simulink model "old_plant_2015B"  (R2015b)
settings: Solver=ode1  StartTime=0.0  StopTime=sim_run  FixedStep=0.001  RelTol=1e-3
InitFcn:
  | [g,m1,T1,f_1s,f_1k,m2,l,f_2k,M_sp,f_1k_lin,f_2k_lin,k1,k2] =...
  |     set_system_parameters();
undefined symbols (not defined in the file): DiscIntNeverNeededParam, f_1k, f_1k_lin, f_1s, f_2k, f_2k_lin, g, k1, k2, l, m1, m2, M_sp, sgn, Standard_Devices, UDP_Protocol, zh_step
libraries: sldrtlib x4, dspnetwork x2
settings Model: Creator=Anony  LastModifiedBy=Anony

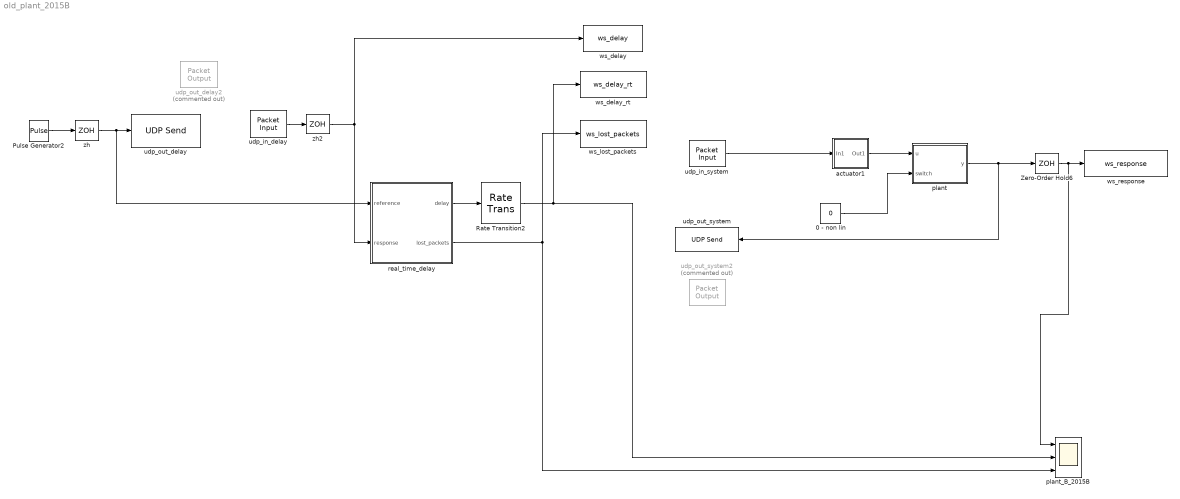
== system old_plant_2015B ==
  0 - non lin : Constant  Value=0
  Pulse Generator2 : DiscretePulseGenerator  PulseType=Time based  Period=0.1
  Rate Transition2 : RateTransition  OutPortSampleTimeOpt=Inherit
  Zero-Order Hold6 : ZeroOrderHold  SampleTime=zh_step
  actuator1 : Subsystem
  plant : Subsystem
  plant_B_2015B : Scope  NumInputPorts=3
  real_time_delay : Subsystem
  udp_in_delay : sldrtlib/Packet Input  SampleTime=0.001  MaxMissedTicks=inf  ShowMissedTicks=off  YieldWhenWaiting=off  DrvName=Standard_Devices/UDP_Protocol  DrvAddress=20000  DrvOptions=[2468394761 20000]  PacketSize=8  DataTypes='double'  ShowReady=off  ShowError=off  PacketID=1  ByteOrder=1  ShowTimestamp=off
      settings: AttributesFormatString=Standard Devices\nUDP Protocol [6982h]
  udp_in_system : sldrtlib/Packet Input  SampleTime=0.001  MaxMissedTicks=inf  ShowMissedTicks=off  YieldWhenWaiting=off  DrvName=Standard_Devices/UDP_Protocol  DrvAddress=20500  DrvOptions=[2468394761 20500]  PacketSize=8  DataTypes='double'  ShowReady=off  ShowError=off  PacketID=1  ByteOrder=1  ShowTimestamp=off
      settings: AttributesFormatString=Standard Devices\nUDP Protocol [6B76h]
  udp_out_delay : dspnetwork/UDP Send  remoteURL='147.32.183.9'  remotePort=21000  localURL='0.0.0.0'  localPortSource=Automatically determine  localPort=27000  sampletime=-1  separateLengthPort=0
  udp_out_delay2 : sldrtlib/Packet Output  Commented=on  SampleTime=0.01  MaxMissedTicks=inf  ShowMissedTicks=off  YieldWhenWaiting=off  DrvName=Standard_Devices/UDP_Protocol  DrvAddress=21000  DrvOptions=[2468394756 21000]  PacketSize=8  DataTypes='double'  ShowReady=off  ShowError=off  PacketID=1  ByteOrder=1  InitialValue=[]  FinalValue=[]
  udp_out_system : dspnetwork/UDP Send  remoteURL='147.32.183.9'  remotePort=21500  localURL='0.0.0.0'  localPortSource=Automatically determine  localPort=27000  sampletime=-1  separateLengthPort=0
  udp_out_system2 : sldrtlib/Packet Output  Commented=on  SampleTime=0.01  MaxMissedTicks=inf  ShowMissedTicks=off  YieldWhenWaiting=off  DrvName=Standard_Devices/UDP_Protocol  DrvAddress=21500  DrvOptions=[2468394761 21500]  PacketSize=8  DataTypes='double'  ShowReady=off  ShowError=off  PacketID=1  ByteOrder=1  InitialValue=[]  FinalValue=[]
  ws_delay : ToWorkspace  VariableName=ws_delay  SaveFormat=Timeseries  SampleTime=zh_step
  ws_delay_rt : ToWorkspace  VariableName=ws_delay_rt  SaveFormat=Timeseries  SampleTime=zh_step
  ws_lost_packets : ToWorkspace  VariableName=ws_lost_packets  SaveFormat=Timeseries  SampleTime=zh_step
  ws_response : ToWorkspace  VariableName=ws_response  SaveFormat=Timeseries  SampleTime=zh_step
  zh : ZeroOrderHold  SampleTime=zh_step
  zh2 : ZeroOrderHold  SampleTime=zh_step
  wires:
  plant/1(y) -> udp_out_system/1, Zero-Order Hold6/1
  0 - non lin/1 -> plant/2(switch)
  actuator1/1(Out1) -> plant/1(u)
  udp_in_system/1 -> actuator1/1(In1)
  udp_in_delay/1 -> zh2/1
  zh2/1 -> real_time_delay/2(response), ws_delay/1
  zh/1 -> udp_out_delay/1, real_time_delay/1(reference)
  real_time_delay/2(lost_packets) -> plant_B_2015B/3, ws_lost_packets/1
  real_time_delay/1(delay) -> Rate Transition2/1
  Pulse Generator2/1 -> zh/1
  Rate Transition2/1 -> ws_delay_rt/1, plant_B_2015B/2
  Zero-Order Hold6/1 -> plant_B_2015B/1, ws_response/1

== system old_plant_2015B/actuator1 ==
  In1 : Inport
  V > N1 : Gain  Gain=4
  mv > V1 : Gain  Gain=1000
  Out1 : Outport
  wires:
  In1/1 -> mv > V1/1
  mv > V1/1 -> V > N1/1
  V > N1/1 -> Out1/1

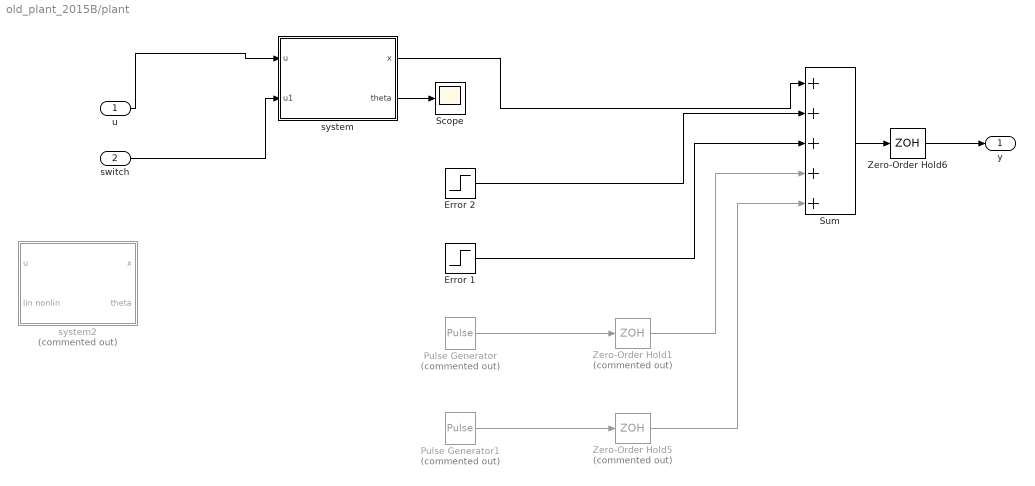
== system old_plant_2015B/plant ==
  u : Inport
  switch : Inport  Port=2
  Error 1 : Step  Time=15  After=0.02  SampleTime=0
  Error 2 : Step  Time=10  After=-0.02  SampleTime=0
  Pulse Generator : DiscretePulseGenerator  Commented=on  PulseType=Time based  Amplitude=0.3  Period=3  PulseWidth=5  PhaseDelay=15
  Pulse Generator1 : DiscretePulseGenerator  Commented=on  PulseType=Time based  Amplitude=-0.18  Period=3  PulseWidth=5  PhaseDelay=25
  Scope : Scope
  Sum : Sum  Inputs=|+++++
  Zero-Order Hold1 : ZeroOrderHold  Commented=on  SampleTime=zh_step
  Zero-Order Hold5 : ZeroOrderHold  Commented=on  SampleTime=zh_step
  Zero-Order Hold6 : ZeroOrderHold  SampleTime=zh_step
  system : Subsystem
  system2 : Subsystem  Commented=on
  y : Outport
  wires:
  system/2(theta) -> Scope/1
  switch/1 -> system/2(u1)
  u/1 -> system/1(u)
  Zero-Order Hold5/1 -> Sum/5
  Pulse Generator1/1 -> Zero-Order Hold5/1
  Zero-Order Hold1/1 -> Sum/4
  Pulse Generator/1 -> Zero-Order Hold1/1
  Error 1/1 -> Sum/3
  system/1(x) -> Sum/1
  Error 2/1 -> Sum/2
  Sum/1 -> Zero-Order Hold6/1
  Zero-Order Hold6/1 -> y/1

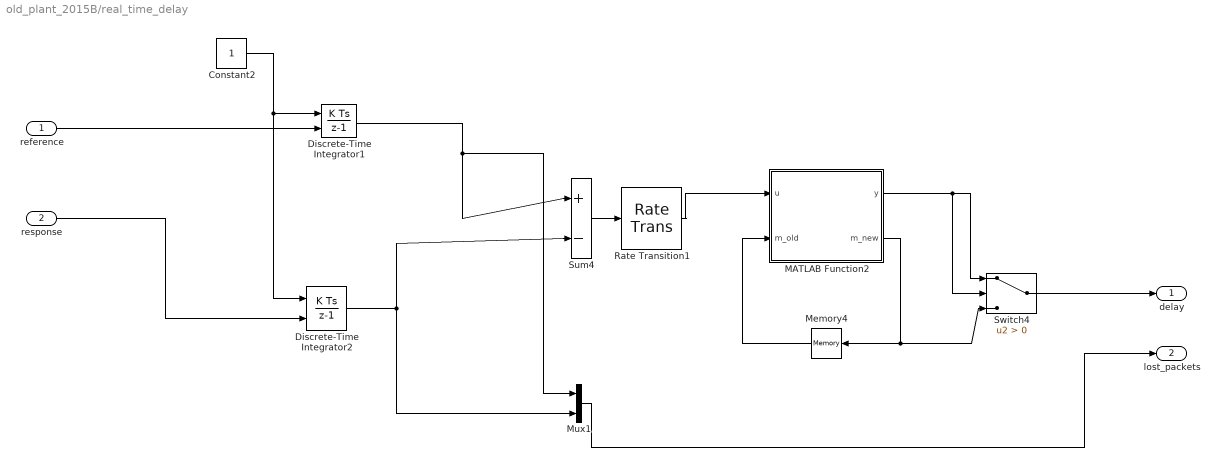
== system old_plant_2015B/real_time_delay ==
  reference : Inport
  response : Inport  Port=2
  Constant2 : Constant
  Discrete-Time Integrator1 : DiscreteIntegrator  ExternalReset=rising  InitialConditionSetting=State (most efficient)  SampleTime=zh_step  ICPrevOutput=DiscIntNeverNeededParam  ICPrevScaledInput=DiscIntNeverNeededParam
  Discrete-Time Integrator2 : DiscreteIntegrator  ExternalReset=rising  InitialConditionSetting=State (most efficient)  SampleTime=zh_step  ICPrevOutput=DiscIntNeverNeededParam  ICPrevScaledInput=DiscIntNeverNeededParam
  MATLAB Function2 : MATLAB Function  TreatAsAtomicUnit=on
  Memory4 : Memory
  Mux1 : Mux  Inputs=2
  Rate Transition1 : RateTransition  OutPortSampleTimeOpt=Inherit
  Sum4 : Sum  Inputs=|+-
  Switch4 : Switch  Criteria=u2 > Threshold
  delay : Outport
  lost_packets : Outport  Port=2
  wires:
  Discrete-Time Integrator1/1 -> Mux1/1, Sum4/1
  reference/1 -> Discrete-Time Integrator1/2
  Constant2/1 -> Discrete-Time Integrator2/1, Discrete-Time Integrator1/1
  response/1 -> Discrete-Time Integrator2/2
  Switch4/1 -> delay/1
  MATLAB Function2/2(m_new) -> Memory4/1, Switch4/3
  Memory4/1 -> MATLAB Function2/2(m_old)
  Discrete-Time Integrator2/1 -> Mux1/2, Sum4/2
  Mux1/1 -> lost_packets/1
  MATLAB Function2/1(y) -> Switch4/2, Switch4/1
  Sum4/1 -> Rate Transition1/1
  Rate Transition1/1 -> MATLAB Function2/1(u)

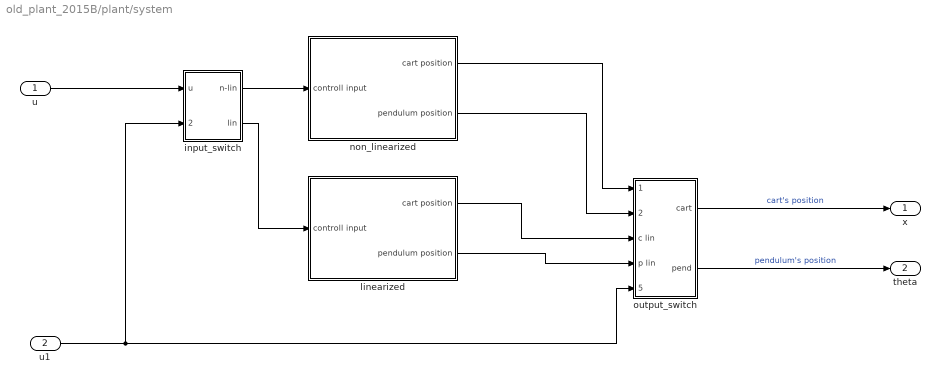
== system old_plant_2015B/plant/system ==
  u : Inport
  u1 : Inport  Port=2
  input_switch : Subsystem
  linearized : Subsystem
  non_linearized : Subsystem
  output_switch : Subsystem
  x : Outport
  theta : Outport  Port=2
  wires:
  u1/1 -> input_switch/2(switch), output_switch/5(switch)
  u/1 -> input_switch/1(u)
  output_switch/2(pend) -> theta/1  "pendulum's position"
  linearized/2("pendulum position ") -> output_switch/4(p lin)
  linearized/1(cart position) -> output_switch/3(c lin)
  non_linearized/2("pendulum position ") -> output_switch/2(p n-lin)
  non_linearized/1(cart position) -> output_switch/1(c n-lin)
  output_switch/1(cart) -> x/1  "cart's position"
  input_switch/2("lin ") -> linearized/1(controll input)
  input_switch/1(n-lin) -> non_linearized/1(controll input)

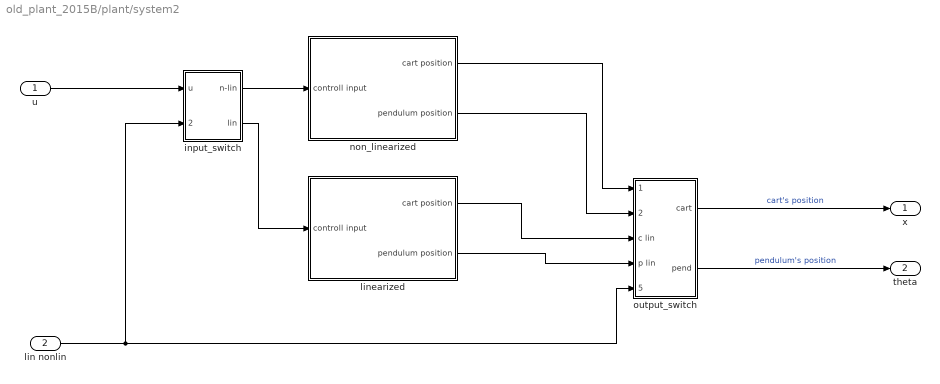
== system old_plant_2015B/plant/system2 ==
  u : Inport
  lin nonlin : Inport  Port=2
  input_switch : Subsystem
  linearized : Subsystem
  non_linearized : Subsystem
  output_switch : Subsystem
  x : Outport
  theta : Outport  Port=2
  wires:
  input_switch/1(n-lin) -> non_linearized/1(controll input)
  input_switch/2("lin ") -> linearized/1(controll input)
  output_switch/1(cart) -> x/1  "cart's position"
  non_linearized/1(cart position) -> output_switch/1(c n-lin)
  non_linearized/2("pendulum position ") -> output_switch/2(p n-lin)
  linearized/1(cart position) -> output_switch/3(c lin)
  linearized/2("pendulum position ") -> output_switch/4(p lin)
  output_switch/2(pend) -> theta/1  "pendulum's position"
  u/1 -> input_switch/1(u)
  lin nonlin/1 -> output_switch/5(switch), input_switch/2(switch)

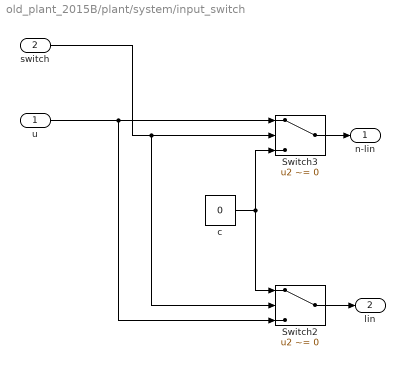
== system old_plant_2015B/plant/system/input_switch ==
  u : Inport
  switch : Inport  Port=2
  Switch2 : Switch  Criteria=u2 ~= 0  Threshold=1
  Switch3 : Switch  Criteria=u2 ~= 0  Threshold=1
  c : Constant  Value=0
  n-lin : Outport
  "lin " : Outport  Port=2
  wires:
  switch/1 -> Switch3/2, Switch2/2
  u/1 -> Switch3/1, Switch2/3
  Switch2/1 -> "lin "/1
  Switch3/1 -> n-lin/1
  c/1 -> Switch2/1, Switch3/3

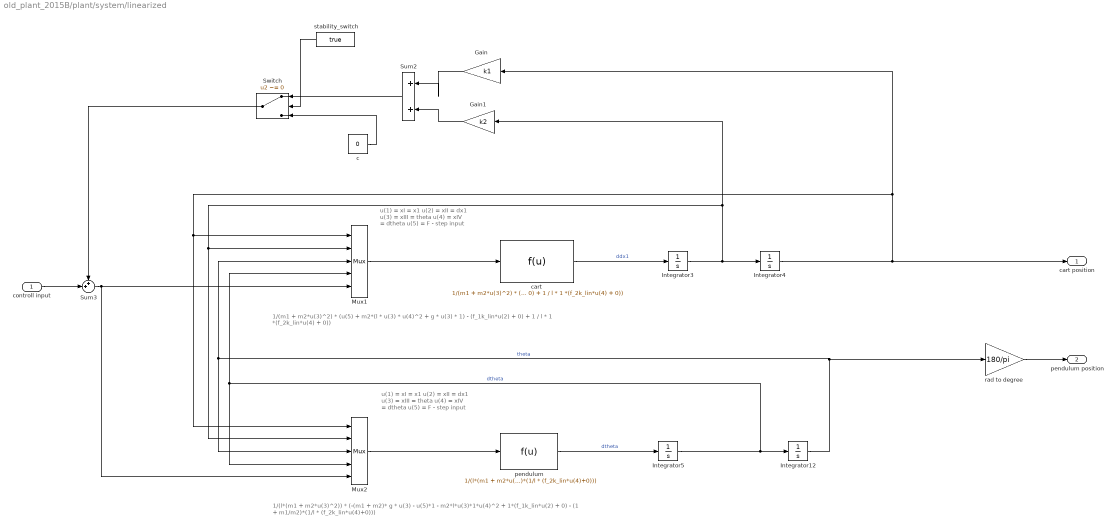
== system old_plant_2015B/plant/system/linearized ==
  note: 1/(l*(m1 + m2*u(3)^2)) * (-(m1 + m2)* g * u(3) - u(5)*1 - m2*l*u(3)*1*u(4)^2 + 1*(f_1k_lin*u(2) + 0) - (1 + m1/m2)*(1/l * (f_2k_lin*u(4)+0)))
  note: 1/(m1 + m2*u(3)^2) * (u(5) + m2*(l * u(3) * u(4)^2 + g * u(3) * 1) - (f_1k_lin*u(2) + 0) + 1 / l * 1 *(f_2k_lin*u(4) + 0))
  note: u(1) = xI = x1
      | u(2) = xII = dx1
      | u(3) = xIII = theta
      | u(4) = xIV = dtheta
      | u(5) = F - step input
  note: u(1) = xI = x1
      | u(2) = xII = dx1
      | u(3) = xIII = theta
      | u(4) = xIV = dtheta
      | u(5) = F - step input
  controll input : Inport
  Gain : Gain  Gain=k1
  Gain1 : Gain  Gain=k2
  Integrator{3..5,12} (4 alike) : Integrator
  Mux1 : Mux  Inputs=5
  Mux2 : Mux  Inputs=5
  Sum2 : Sum  Inputs=|++
  Sum3 : Sum  Inputs=++|
  Switch : Switch  Criteria=u2 ~= 0
  c : Constant  Value=0
  cart : Fcn  Expr=1/(m1 + m2*u(3)^2) * (u(5) + m2*(l * u(3) * u(4)^2 + g * u(3) * 1) - (f_1k_lin*u(2) + 0) + 1 / l * 1 *(f_2k_lin*u(4) + 0))
  "pendulum " : Fcn  Expr=1/(l*(m1 + m2*u(3)^2)) * (-(m1 + m2)* g * u(3) - u(5)*1 - m2*l*u(3)*1*u(4)^2 + 1*(f_1k_lin*u(2) + 0) - (1 + m1/m2)*(1/l * (f_2k_lin*u(4)+0)))
  rad to degree : Gain  Gain=180/pi
  stability_switch : Constant  Value=true
  cart position : Outport
  "pendulum position " : Outport  Port=2
  wires:
  stability_switch/1 -> Switch/2
  Switch/1 -> Sum3/1
  Sum2/1 -> Switch/1
  Sum3/1 -> Mux1/5, Mux2/5
  controll input/1 -> Sum3/2
  Gain1/1 -> Sum2/2
  Gain/1 -> Sum2/1
  Integrator4/1 -> cart position/1, Mux2/1, Mux1/1, Gain/1
  Integrator3/1 -> Integrator4/1, Mux2/2, Mux1/2, Gain1/1
  cart/1 -> Integrator3/1  "ddx1"
  Mux2/1 -> "pendulum "/1
  "pendulum "/1 -> Integrator5/1  "dtheta"
  Integrator5/1 -> Integrator12/1, Mux1/4, Mux2/4  "dtheta"
  Integrator12/1 -> rad to degree/1, Mux1/3, Mux2/3  "theta"
  Mux1/1 -> cart/1
  rad to degree/1 -> "pendulum position "/1
  c/1 -> Switch/3

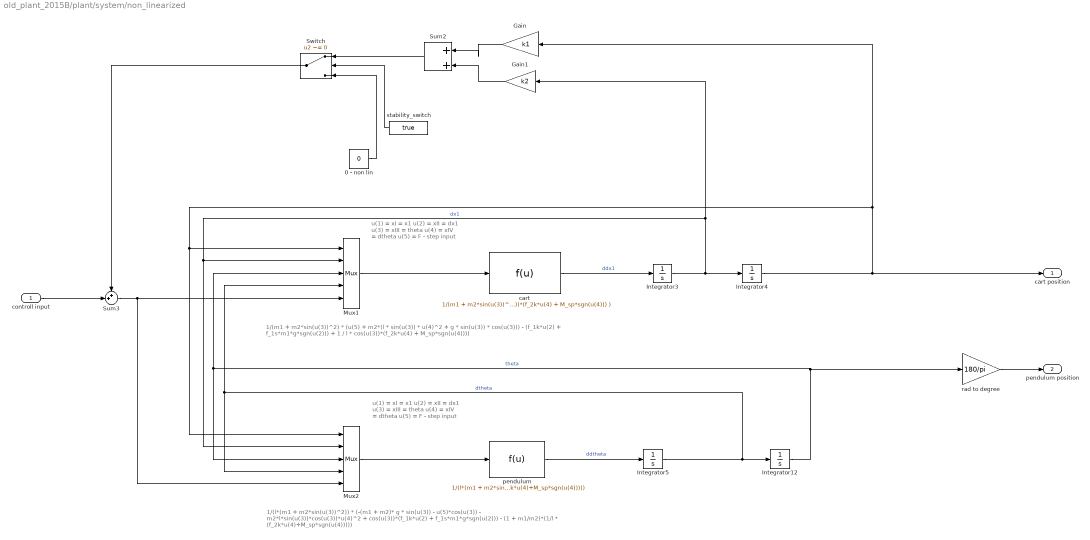
== system old_plant_2015B/plant/system/non_linearized ==
  note: u(1) = xI = x1
      | u(2) = xII = dx1
      | u(3) = xIII = theta
      | u(4) = xIV = dtheta
      | u(5) = F - step input
  note: u(1) = xI = x1
      | u(2) = xII = dx1
      | u(3) = xIII = theta
      | u(4) = xIV = dtheta
      | u(5) = F - step input
  note: 1/(m1 + m2*sin(u(3))^2) * (u(5) + m2*(l * sin(u(3)) * u(4)^2 + g * sin(u(3)) * cos(u(3))) - (f_1k*u(2) + f_1s*m1*g*sgn(u(2))) + 1 / l * cos(u(3))*(f_2k*u(4) + M_sp*sgn(u(4))))
  note: 1/(l*(m1 + m2*sin(u(3))^2)) * (-(m1 + m2)* g * sin(u(3)) - u(5)*cos(u(3)) - m2*l*sin(u(3))*cos(u(3))*u(4)^2 + cos(u(3))*(f_1k*u(2) + f_1s*m1*g*sgn(u(2))) - (1 + m1/m2)*(1/l * (f_2k*u(4)+M_sp*sgn(u(4)))))
  controll input : Inport
  0 - non lin : Constant  Value=0
  Gain : Gain  Gain=k1
  Gain1 : Gain  Gain=k2
  Integrator{3..5,12} (4 alike) : Integrator
  Mux1 : Mux  Inputs=5
  Mux2 : Mux  Inputs=5
  Sum2 : Sum  Inputs=|++
  Sum3 : Sum  Inputs=++|
  Switch : Switch  Criteria=u2 ~= 0
  cart : Fcn  Expr=1/(m1 + m2*sin(u(3))^2) * (u(5) + m2*(l * sin(u(3)) * u(4)^2 + g * sin(u(3)) * cos(u(3))) - (f_1k*u(2) + f_1s*m1*g*sgn(u(2))) + 1 / l * cos(u(3))*(f_2k*u(4) + M_sp*sgn(u(4))) )
  "pendulum " : Fcn  Expr=1/(l*(m1 + m2*sin(u(3))^2)) * (-(m1 + m2)* g * sin(u(3)) - u(5)*cos(u(3)) - m2*l*sin(u(3))*cos(u(3))*u(4)^2 + cos(u(3))*(f_1k*u(2) + f_1s*m1*g*sgn(u(2))) - (1 + m1/m2)*(1/l * (f_2k*u(4)+M_sp*sgn(u(4)))))
  rad to degree : Gain  Gain=180/pi
  stability_switch : Constant  Value=true
  cart position : Outport
  "pendulum position " : Outport  Port=2
  wires:
  Sum3/1 -> Mux1/5, Mux2/5
  controll input/1 -> Sum3/2
  stability_switch/1 -> Switch/2
  Switch/1 -> Sum3/1
  Sum2/1 -> Switch/1
  Gain1/1 -> Sum2/2
  Gain/1 -> Sum2/1
  Integrator4/1 -> Mux1/1, Mux2/1, Gain/1, cart position/1
  rad to degree/1 -> "pendulum position "/1
  Mux1/1 -> cart/1
  Integrator12/1 -> Mux2/3, Mux1/3, rad to degree/1  "theta"
  Integrator3/1 -> Mux1/2, Mux2/2, Gain1/1, Integrator4/1  "dx1"
  Integrator5/1 -> Mux2/4, Mux1/4, Integrator12/1  "dtheta"
  "pendulum "/1 -> Integrator5/1  "ddtheta"
  Mux2/1 -> "pendulum "/1
  cart/1 -> Integrator3/1  "ddx1"
  0 - non lin/1 -> Switch/3

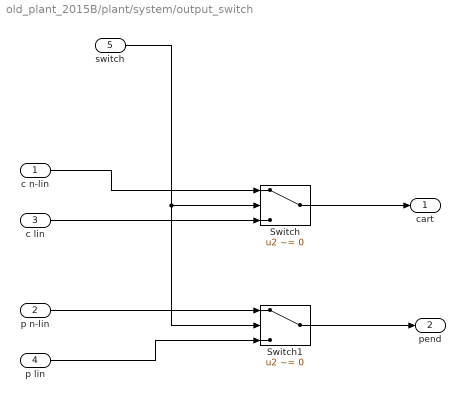
== system old_plant_2015B/plant/system/output_switch ==
  c n-lin : Inport
  p n-lin : Inport  Port=2
  c lin : Inport  Port=3
  p lin : Inport  Port=4
  switch : Inport  Port=5
  Switch : Switch  Criteria=u2 ~= 0  Threshold=1
  Switch1 : Switch  Criteria=u2 ~= 0  Threshold=1
  cart : Outport
  pend : Outport  Port=2
  wires:
  p n-lin/1 -> Switch1/1
  c n-lin/1 -> Switch/1
  Switch1/1 -> pend/1
  c lin/1 -> Switch/3
  Switch/1 -> cart/1
  p lin/1 -> Switch1/3
  switch/1 -> Switch/2, Switch1/2

== system old_plant_2015B/plant/system2/input_switch ==
  u : Inport
  switch : Inport  Port=2
  Constant : Constant  Value=0
  Switch2 : Switch  Criteria=u2 ~= 0  Threshold=1
  Switch3 : Switch  Criteria=u2 ~= 0  Threshold=1
  n-lin : Outport
  "lin " : Outport  Port=2
  wires:
  Switch3/1 -> n-lin/1
  Switch2/1 -> "lin "/1
  u/1 -> Switch2/3, Switch3/1
  switch/1 -> Switch2/2, Switch3/2
  Constant/1 -> Switch2/1, Switch3/3

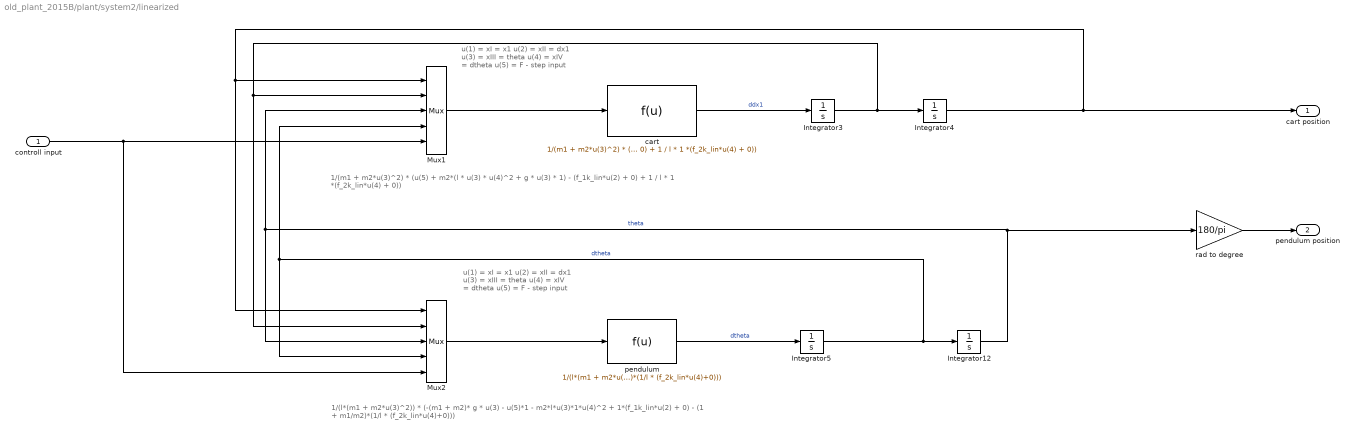
== system old_plant_2015B/plant/system2/linearized ==
  note: u(1) = xI = x1
      | u(2) = xII = dx1
      | u(3) = xIII = theta
      | u(4) = xIV = dtheta
      | u(5) = F - step input
  note: u(1) = xI = x1
      | u(2) = xII = dx1
      | u(3) = xIII = theta
      | u(4) = xIV = dtheta
      | u(5) = F - step input
  note: 1/(m1 + m2*u(3)^2) * (u(5) + m2*(l * u(3) * u(4)^2 + g * u(3) * 1) - (f_1k_lin*u(2) + 0) + 1 / l * 1 *(f_2k_lin*u(4) + 0))
  note: 1/(l*(m1 + m2*u(3)^2)) * (-(m1 + m2)* g * u(3) - u(5)*1 - m2*l*u(3)*1*u(4)^2 + 1*(f_1k_lin*u(2) + 0) - (1 + m1/m2)*(1/l * (f_2k_lin*u(4)+0)))
  controll input : Inport
  Integrator{3..5,12} (4 alike) : Integrator
  Mux1 : Mux  Inputs=5
  Mux2 : Mux  Inputs=5
  cart : Fcn  Expr=1/(m1 + m2*u(3)^2) * (u(5) + m2*(l * u(3) * u(4)^2 + g * u(3) * 1) - (f_1k_lin*u(2) + 0) + 1 / l * 1 *(f_2k_lin*u(4) + 0))
  "pendulum " : Fcn  Expr=1/(l*(m1 + m2*u(3)^2)) * (-(m1 + m2)* g * u(3) - u(5)*1 - m2*l*u(3)*1*u(4)^2 + 1*(f_1k_lin*u(2) + 0) - (1 + m1/m2)*(1/l * (f_2k_lin*u(4)+0)))
  rad to degree : Gain  Gain=180/pi
  cart position : Outport
  "pendulum position " : Outport  Port=2
  wires:
  rad to degree/1 -> "pendulum position "/1
  Mux1/1 -> cart/1
  Integrator12/1 -> Mux2/3, Mux1/3, rad to degree/1  "theta"
  Integrator5/1 -> Mux2/4, Mux1/4, Integrator12/1  "dtheta"
  "pendulum "/1 -> Integrator5/1  "dtheta"
  Mux2/1 -> "pendulum "/1
  cart/1 -> Integrator3/1  "ddx1"
  Integrator3/1 -> Mux1/2, Mux2/2, Integrator4/1
  Integrator4/1 -> Mux1/1, Mux2/1, cart position/1
  controll input/1 -> Mux2/5, Mux1/5

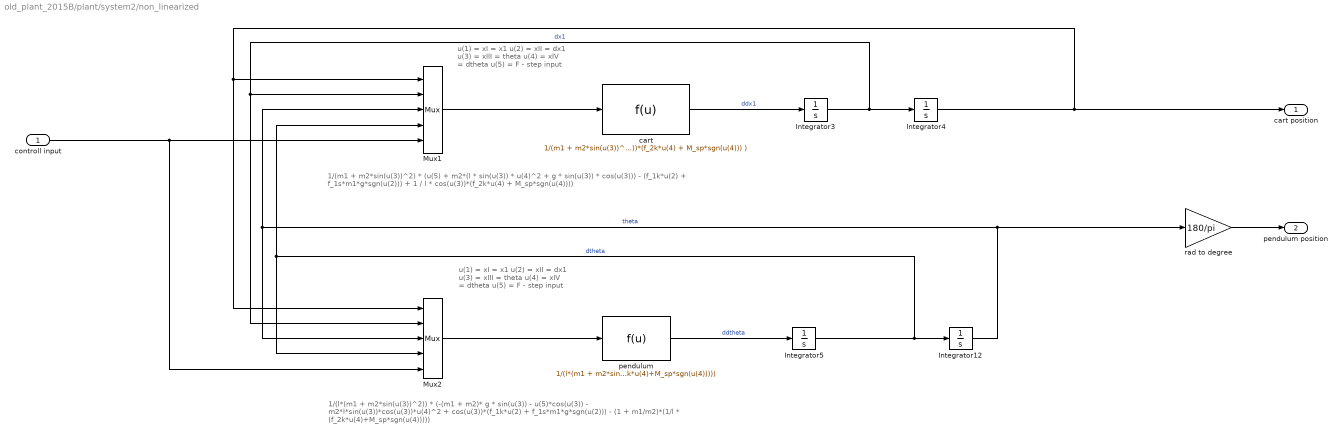
== system old_plant_2015B/plant/system2/non_linearized ==
  note: 1/(l*(m1 + m2*sin(u(3))^2)) * (-(m1 + m2)* g * sin(u(3)) - u(5)*cos(u(3)) - m2*l*sin(u(3))*cos(u(3))*u(4)^2 + cos(u(3))*(f_1k*u(2) + f_1s*m1*g*sgn(u(2))) - (1 + m1/m2)*(1/l * (f_2k*u(4)+M_sp*sgn(u(4)))))
  note: 1/(m1 + m2*sin(u(3))^2) * (u(5) + m2*(l * sin(u(3)) * u(4)^2 + g * sin(u(3)) * cos(u(3))) - (f_1k*u(2) + f_1s*m1*g*sgn(u(2))) + 1 / l * cos(u(3))*(f_2k*u(4) + M_sp*sgn(u(4))))
  note: u(1) = xI = x1
      | u(2) = xII = dx1
      | u(3) = xIII = theta
      | u(4) = xIV = dtheta
      | u(5) = F - step input
  note: u(1) = xI = x1
      | u(2) = xII = dx1
      | u(3) = xIII = theta
      | u(4) = xIV = dtheta
      | u(5) = F - step input
  controll input : Inport
  Integrator{3..5,12} (4 alike) : Integrator
  Mux1 : Mux  Inputs=5
  Mux2 : Mux  Inputs=5
  cart : Fcn  Expr=1/(m1 + m2*sin(u(3))^2) * (u(5) + m2*(l * sin(u(3)) * u(4)^2 + g * sin(u(3)) * cos(u(3))) - (f_1k*u(2) + f_1s*m1*g*sgn(u(2))) + 1 / l * cos(u(3))*(f_2k*u(4) + M_sp*sgn(u(4))) )
  "pendulum " : Fcn  Expr=1/(l*(m1 + m2*sin(u(3))^2)) * (-(m1 + m2)* g * sin(u(3)) - u(5)*cos(u(3)) - m2*l*sin(u(3))*cos(u(3))*u(4)^2 + cos(u(3))*(f_1k*u(2) + f_1s*m1*g*sgn(u(2))) - (1 + m1/m2)*(1/l * (f_2k*u(4)+M_sp*sgn(u(4)))))
  rad to degree : Gain  Gain=180/pi
  cart position : Outport
  "pendulum position " : Outport  Port=2
  wires:
  cart/1 -> Integrator3/1  "ddx1"
  Mux2/1 -> "pendulum "/1
  "pendulum "/1 -> Integrator5/1  "ddtheta"
  Integrator5/1 -> Integrator12/1, Mux1/4, Mux2/4  "dtheta"
  Integrator3/1 -> Integrator4/1, Mux2/2, Mux1/2  "dx1"
  Integrator12/1 -> rad to degree/1, Mux1/3, Mux2/3  "theta"
  Mux1/1 -> cart/1
  rad to degree/1 -> "pendulum position "/1
  Integrator4/1 -> cart position/1, Mux2/1, Mux1/1
  controll input/1 -> Mux2/5, Mux1/5

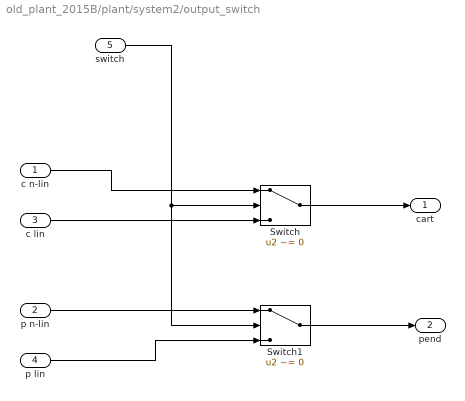
== system old_plant_2015B/plant/system2/output_switch ==
  c n-lin : Inport
  p n-lin : Inport  Port=2
  c lin : Inport  Port=3
  p lin : Inport  Port=4
  switch : Inport  Port=5
  Switch : Switch  Criteria=u2 ~= 0  Threshold=1
  Switch1 : Switch  Criteria=u2 ~= 0  Threshold=1
  cart : Outport
  pend : Outport  Port=2
  wires:
  switch/1 -> Switch1/2, Switch/2
  p lin/1 -> Switch1/3
  Switch/1 -> cart/1
  c lin/1 -> Switch/3
  Switch1/1 -> pend/1
  c n-lin/1 -> Switch/1
  p n-lin/1 -> Switch1/1

== matlab function old_plant_2015B/real_time_delay/MATLAB Function2 ==
  data: u input; y output; m_new output; m_old input
function [y,m_new] = fcn(u,m_old)
%#codegen
if(u>0)
    y = u;
    m_new = u;
else
    y =0;
    m_new = m_old;
end
